simulink model "PassiveCWSsystem"  (R2016b)
settings: Solver=FixedStepAuto  StartTime=0.0  StopTime=10.0  FixedStep=0.1  RelTol=1e-3  EnableMultiTasking=on
settings Model: Creator=Josef  LastModifiedBy=NEATdemo
settings OptimizationCC: LifeSpan=inf
settings DebuggingCC: SFUnexpectedBacktrackingDiag=warning  SFNoUnconditionalDefaultTransitionDiag=warning  SFExecutionAtInitializationDiag=none
settings GRTTargetCC: TargetLangStandard=C89/C90 (ANSI)
settings ConfigComp: CovMetricSettings=dw  CovHtmlReporting=on  CovSaveCumulativeToWorkspaceVar=on  CovSaveSingleToWorkspaceVar=on  CovExternalEMLEnable=off

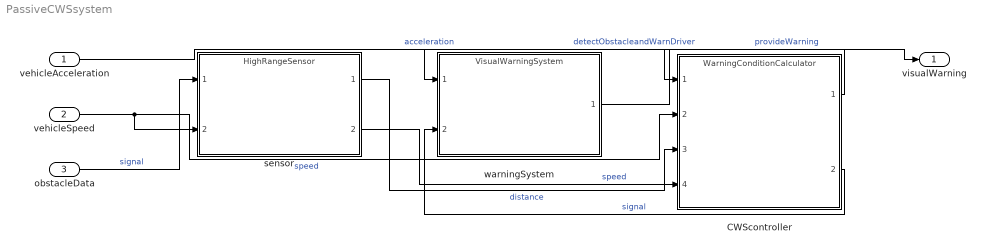
== system PassiveCWSsystem ==
  vehicleAcceleration : Inport
      settings: AttributesFormatString=acceleration
  vehicleSpeed : Inport  Port=2
      settings: AttributesFormatString=speed
  obstacleData : Inport  Port=3
      settings: AttributesFormatString=signal
  CWScontroller : ModelReference  ModelNameDialog=WarningConditionCalculator  SimulationMode=Normal  ModelReferenceVersion=1.9
  sensor : ModelReference  ModelNameDialog=HighRangeSensor  SimulationMode=Normal  ModelReferenceVersion=1.3
  warningSystem : ModelReference  ModelNameDialog=VisualWarningSystem  SimulationMode=Normal  ModelReferenceVersion=1.10
  visualWarning : Outport
      settings: AttributesFormatString=provideWarning
  wires:
  CWScontroller/2 -> warningSystem/2  "signal"
  CWScontroller/1 -> warningSystem/1  "detectObstacleandWarnDriver"
  sensor/1 -> CWScontroller/3  "distance"
  sensor/2 -> CWScontroller/4  "speed"
  warningSystem/1 -> visualWarning/1  "provideWarning"
  vehicleAcceleration/1 -> CWScontroller/1  "acceleration"
  vehicleSpeed/1 -> sensor/2, CWScontroller/2  "speed"
  obstacleData/1 -> sensor/1  "signal"
